simulink subsystem "PvtSubSys_PLAN_AP"  (R2020b)
settings: Solver=VariableStepAuto  StartTime=0.0  StopTime=10.0  RelTol=1e-3
undefined symbols (not defined in the file or in its folder): C_LongCtrl_0_Single, C_LongCtrl_0_Uint8, C_LongCtrl_Mph2Kph, magnitude, P_LongCtrl_accelTargAbsThrd, P_LongCtrl_AddVelAccelChange, P_LongCtrl_AddVelAccelThrd, P_LongCtrl_AddVelDistDesThrd, P_LongCtrl_AddVelEnable, P_LongCtrl_AddVelRefMsThrd, P_LongCtrl_ALaLowerChar, P_LongCtrl_ALaUpperCharEco, P_LongCtrl_ALaUpperCharNormal, P_LongCtrl_ALaUpperCharSport, P_LongCtrl_ALCAccLimitByDangerXAxis, P_LongCtrl_ALCAccLimitByDangerYAxis, P_LongCtrl_ALvAcceleLowerChar, P_LongCtrl_ALvAcceleUpperCharEco, P_LongCtrl_ALvAcceleUpperCharNormal, P_LongCtrl_ALvAcceleUpperCharSport, P_LongCtrl_CCaccelCCNeg2PosJerk, P_LongCtrl_CCaccelCCPosJerk, P_LongCtrl_CCaccelLowerIsLaneChange, P_LongCtrl_CCaccelMaxLCActive, P_LongCtrl_CCaccelMinECOAL, P_LongCtrl_CCaccelMinFastDecel, P_LongCtrl_CCaccelMinNoFastDecel, P_LongCtrl_CCaccelMinNormAL, P_LongCtrl_CCaccelMinSportAL, P_LongCtrl_CCaccelUpperCC, P_LongCtrl_CCaccelUpperCCSafeStop, P_LongCtrl_CCaMinNegAcceleLowerBand, P_LongCtrl_CCaMinNegAcceleUpperBand, P_LongCtrl_CCaMinPosAcceleLowerBand, P_LongCtrl_CCaMinPosAcceleUpperBand, P_LongCtrl_CCbECO, P_LongCtrl_CCbNorm, P_LongCtrl_CCbSport, P_LongCtrl_CCcoefESPSpd2IPSpd1, P_LongCtrl_CCcoefESPSpd2IPSpd2, P_LongCtrl_CCdecelCCJerk, P_LongCtrl_CCdecelCCJerkNegVLCInternalAcc, P_LongCtrl_CCfacNegAcceleLowerBand, P_LongCtrl_CCfacNegAcceleUpperBand, P_LongCtrl_CCfacPosAcceleLowerBand, P_LongCtrl_CCfacPosAcceleUpperBand, P_LongCtrl_CCkECO, P_LongCtrl_CCkNorm, P_LongCtrl_CCkSport, P_LongCtrl_CCLCIncSetSpdAdd, P_LongCtrl_CCLCIncSetSpdAddCntStartValue, P_LongCtrl_CCResumeDelayDeltaVel, P_LongCtrl_CCtAcceleTimeNeg, P_LongCtrl_CCtAcceleTimeNegCorrXAxis, P_LongCtrl_CCtAcceleTimeNegCorrYAxis, P_LongCtrl_CCtAcceleTimePos, P_LongCtrl_CCtAcceleTimePosCorrXAxis, P_LongCtrl_CCtAcceleTimePosCorrYAxis, P_LongCtrl_CCtStepVelPlan, P_LongCtrl_CCtTotVelPlan ... (+150)
libraries: simulink x62, TrueDurationTime x1
(part 6 of 7)

== stateflow chart PvtSubSys_PLAN_AP/AP/AP/IC/CurvatureOfMapCalc/Chart ==
  state velSubjLimMap = velSubjLimChar(LongCtrl_IC_EHRV2_CurMatrixLP) [function]
  state velDelta = velDeltaCalc(velSubjLimMap,velSubj) [function]
  state accelICCurvatureMapMatrix = accelICCurvatureMapPosCalc(velDelta) [function]
  state accelICCurvatureMapMatrix = accelICCurvatureMapNegCalc(velDelta) [function]
  state accelICCurvatureMapMatrix = accelICCurvatureMapDistExceed(LongCtrl_IC_EHRV2_CurDisMatrix,velDelta) [function]
  state distDesCurvatureMap = distDesCurvatureMapCalc(velDelta,accelICCurvatureMapMatrix) [function]
  (default) -> (junction 1)
  (junction 1) -> (junction 6) [order 1] : [LongCtrl_IC_EHRV2_CurMatrixSize>0&&(min(LongCtrl_IC_EHRV2_CurMatrixLP)<0.15)]
  (junction 1) -> (junction 10) [order 2] : {accelICCurvatureMapMatrix=repmat(single(16),1,10);}
  (junction 6) -> (junction 8) : {velSubjLimMap = velSubjLimChar(LongCtrl_IC_EHRV2_CurMatrixLP);
      |  velDelta = velDeltaCalc(velSubjLimMap,velSubj);
      |  accelICCurvatureMapMatrix=repmat(single(16),1,10);
      |  distDesCurvatureMap=repmat(single(500),1,10);
      |  i=uint8(1);}
  (junction 8) -> (junction 13) [order 1] : [i<=LongCtrl_IC_EHRV2_CurMatrixSize&&...
      |  abs(LongCtrl_IC_EHRV2_CurMatrixLP(1,i))<0.15]
  (junction 91) -> (junction 8) : {i=i+uint8(1);}
  (junction 8) -> (junction 36) [order 2]
  (junction 13) -> (junction 69)
  (junction 69) -> (junction 70) [order 1] : [velDelta(i)>0]
  (junction 69) -> (junction 55) [order 2] : {accelICCurvatureMapMatrix(1,i) = accelICCurvatureMapNegCalc(velDelta(1,i));
      |  distDesCurvatureMap(1,i) = distDesCurvatureMapCalc(velDelta(1,i),accelICCurvatureMapMatrix(1,i));}
  (junction 70) -> (junction 73) : {accelICCurvatureMapMatrix(1,i) = accelICCurvatureMapPosCalc(velDelta(1,i));}
  (junction 55) -> (junction 56) [order 1] : [distDesCurvatureMap(1,i)>LongCtrl_IC_EHRV2_CurDisMatrix(1,i)]
  (junction 55) -> (junction 57) [order 2] : {accelICCurvatureMapMatrix(1,i) =single(0.5);}
  (junction 56) -> (junction 58) : {accelICCurvatureMapMatrix(1,i) = accelICCurvatureMapDistExceed(LongCtrl_IC_EHRV2_CurDisMatrix(1,i),velDelta(1,i));
      |  accelICCurvatureMapMatrix(1,i) =max(single(-3.5),accelICCurvatureMapMatrix(1,i));}
  (junction 58) -> (junction 57)
  (junction 57) -> (junction 91)
  (junction 73) -> (junction 91)
  (junction 36) -> (junction 10)
  (junction 10) -> (junction 103) : {accelICCurvatureMapMin=min(accelICCurvatureMapMatrix);}
  (junction 103) -> (junction 107) [order 1] : [accelICCurvatureMapMin>0]
  (junction 103) -> (junction 111) [order 2] : {accelDesCurvatureMap=accelICCurvatureMapMin;}
  (junction 107) -> (junction 109) : {accelDesCurvatureMap=accelICCurvatureMapMatrix(1);}
  (junction 109) -> (junction 111)
  (junction 111) -> (junction 114)
  (junction 114) -> (junction 117) [order 1] : [P_LongCtrl_IC_EHRV2Enable==0]
  (junction 114) -> (junction 121) [order 2]
  (junction 117) -> (junction 119) : {accelDesCurvatureMap=single(16);}
  (junction 119) -> (junction 121)
  (junction 121) -> (junction 124)
  data: LongCtrl_IC_EHRV2_CurMatrixLP function_input single size=[1 10]; velSubjLimMap function_output; velSubjLimMap function_input single size=[1 10]; velSubj function_input single size=1; velDelta function_output; velDelta function_input single size=1; accelICCurvatureMapMatrix function_output; velDelta function_input single size=1; accelICCurvatureMapMatrix function_output; LongCtrl_IC_EHRV2_CurDisMatrix function_input single size=1; accelICCurvatureMapMatrix function_output; velDelta function_input single size=1; velDelta function_input single size=1; accelICCurvatureMapMatrix function_input single size=1; distDesCurvatureMap function_output; LongCtrl_IC_EHRV2_CurMatrixLP input single size=[1,10]; LongCtrl_IC_EHRV2_CurDisMatrix input single size=[1,10]; LongCtrl_IC_EHRV2_CurMatrixSize input uint8; velSubj input single; i local uint8; velSubjLimMap local single size=[1,10]; accelICCurvatureMapMatrix output single size=[1,10]; velDelta local single size=[1,10]; accelICCurvatureMapMin local single; distDesCurvatureMap output single size=[1,10]; accelDesCurvatureMap output single; P_LongCtrl_IC_EHRV2Enable parameter boolean

== stateflow chart PvtSubSys_PLAN_AP/AP/AP/IC/CurvatureOfRoadCalc/If Action Subsystem/For Each Subsystem/CurvatureChar ==
  state Curvature1 = Curvature1Calc(GetL1dC2V,GetL1dC3V,GetR1dC2V,GetR1dC3V,GetL1dDisFront,GetR1dDisFront,velSubj) [function]
  state Curvature2 = Curvature2Calc(GetL1dC2V,GetL1dC3V,GetL1dDisFront,velSubj) [function]
  state Curvature3 = Curvature3Calc(GetR1dC2V,GetR1dC3V,GetR1dDisFront,velSubj) [function]
  (default) -> (junction 10)
  (junction 10) -> (junction 12) [order 1] : [(L1bIsLineExist==1)&&(R1bIsLineExis==1)]
  (junction 10) -> (junction 11) [order 2]
  (junction 12) -> (junction 17) : {Curvature1 = Curvature1Calc(GetL1dC2V,GetL1dC3V,GetR1dC2V,GetR1dC3V,GetL1dDisFront,GetR1dDisFront,velSubj);
      |  CurvatureIFC=Curvature1;}
  (junction 11) -> (junction 29) [order 1] : [(L1bIsLineExist==1)&&(R1bIsLineExis!=1)]
  (junction 11) -> (junction 27) [order 2]
  (junction 29) -> (junction 36) : {Curvature2 = Curvature2Calc(GetL1dC2V,GetL1dC3V,GetL1dDisFront,velSubj);
      |  CurvatureIFC=Curvature2;}
  (junction 27) -> (junction 40) [order 1] : [(L1bIsLineExist!=1)&&(R1bIsLineExis==1)]
  (junction 27) -> (junction 38) [order 2] : {CurvatureIFC=single(0);}
  (junction 40) -> (junction 42) : {Curvature3 = Curvature3Calc(GetR1dC2V,GetR1dC3V,GetR1dDisFront,velSubj);
      |  CurvatureIFC=Curvature3;}
  data: GetL1dC2V function_input; GetL1dC3V function_input; GetR1dC2V function_input; GetR1dC3V function_input; GetL1dDisFront function_input; GetR1dDisFront function_input; Curvature1 function_output; velSubj function_input; GetL1dC2V function_input; GetL1dC3V function_input; GetL1dDisFront function_input; Curvature2 function_output; velSubj function_input; GetR1dC2V function_input; GetR1dC3V function_input; GetR1dDisFront function_input; Curvature3 function_output; velSubj function_input; L1bIsLineExist input boolean; R1bIsLineExis input boolean; CurvatureIFC output single; Curvature1 local double; Curvature2 local double; Curvature3 local double; GetL1dC2V input; GetL1dC3V input; GetL1dDisFront input; GetR1dC2V input; GetR1dC3V input; GetR1dDisFront input; velSubj input

== matlab function PvtSubSys_PLAN_AP/AP/AP/IC/Subsystem1/CalcEgoVehMove ==
  data: dDeltaX output single size=1; tCycle input single size=1; Kap input single size=1; velSubj input single size=1; dDeltaY output single size=1; CosOfPsi output single size=1; SinOfPsi output single size=1
function [dDeltaX,dDeltaY,CosOfPsi,SinOfPsi] = EgoVehicleMovement(tCycle,Kap,velSubj)
%#codegen
if Kap==0
    dDeltaX = velSubj*tCycle;
    dDeltaY = single(0);
    CosOfPsi = single(1);
    SinOfPsi = single(0);
else
    t_Psi = Kap*velSubj*tCycle;
    SinOfPsi = sin(t_Psi);
    CosOfPsi = cos(t_Psi);
    dDeltaX = SinOfPsi/Kap;
    dDeltaY = 2*(sin(t_Psi/2)*sin(t_Psi/2))/Kap;
end

== matlab function PvtSubSys_PLAN_AP/AP/AP/IC/Subsystem1/KeepLane ==
  data: KeepLineSts output; P_LongCtrl_KeepLaneTime input; P_LongCtrl_KeepLaneSurDis input; tCycle input single; velSubj input; Cur_LineValid input boolean; Cur_A3 input single; Cur_A2 input single; Cur_A1 input single; Cur_A0 input single; Cur_dDisFront input single; LineUpdate input boolean; dDeltaX input single; dDeltaY input single; CosOfPsi input single; SinOfPsi input single; LineValidK1 input boolean; A3K1 input single; A2K1 input single; A1K1 input single; A0K1 input single; dDisFrontK1 input single; tLostK1 input single; LineValid output boolean; A3 output single; A2 output single; A1 output single; A0 output single; dDisFront output single; tLost output single
function [KeepLineSts,LineValid,A3,A2,A1,A0,dDisFront,tLost] = ...
    VisFilter(P_LongCtrl_KeepLaneTime,P_LongCtrl_KeepLaneSurDis,...
    tCycle,velSubj,Cur_LineValid,Cur_A3,Cur_A2,Cur_A1,Cur_A0,Cur_dDisFront,LineUpdate,...
    dDeltaX,dDeltaY,CosOfPsi,SinOfPsi,...
    LineValidK1,A3K1,A2K1,A1K1,A0K1,dDisFrontK1,tLostK1)

A3 = single(zeros(2,1));
A2 = single(zeros(2,1));
A1 = single(zeros(2,1));
A0 = single(zeros(2,1));
dDisFront = single(zeros(2,1));
tLost = single(zeros(2,1));
LineValid = false(2,1);
KeepLineSts = uint8(zeros(2,1));
for i=1:1:2
    if (Cur_LineValid(i)==true)&&(LineUpdate==true)
        LineValid(i) = true;
        A3(i) = Cur_A3(i);
        A2(i) = Cur_A2(i);
        A1(i) = Cur_A1(i);
        A0(i) = Cur_A0(i);
        dDisFront(i) = Cur_dDisFront(i);
        tLost(i) = single(0);
        KeepLineSts(i) = uint8(0);
    else
        tLost(i) = min(tLostK1(i) + tCycle,single(10));
        if (LineValidK1(i)==true)&&(tLost(i)<P_LongCtrl_KeepLaneTime)
            xi = [0;0.25*dDisFrontK1(i);0.5*dDisFrontK1(i);dDisFrontK1(i)];
            yi = A3K1(i)*xi.^3 + A2K1(i)*xi.^2 + A1K1(i)*xi + A0K1(i);
            t_dx = xi-dDeltaX;
            t_dy = yi-dDeltaY;
            TmpX = t_dx*CosOfPsi+t_dy*SinOfPsi;
            TmpY = -t_dx*SinOfPsi+t_dy*CosOfPsi;
            [A3(i),A2(i),A1(i),A0(i)] = pl(TmpX,TmpY);
            LineValid(i) = true;
            dDisFront(i) = dDisFrontK1(i) - velSubj*tCycle;
            if dDisFront(i)<P_LongCtrl_KeepLaneSurDis
                LineValid(i) = false;
                KeepLineSts(i) = uint8(1);
            else
                KeepLineSts(i) = uint8(2);
            end
        else
            LineValid(i) = false;
            A3(i) = single(0);
            A2(i) = single(0);
            A1(i) = single(0);
            A0(i) = single(0);
            dDisFront(i) = single(0);
            KeepLineSts(i) = uint8(3);
        end
    end
end

== matlab function PvtSubSys_PLAN_AP/AP/AP/IC/Subsystem1/LineFilter ==
  data: P_LongCtrl_LaneAvailStd input; P_LongCtrl_LaneAvailStdMax input; P_LongCtrl_LaneAvailStdAverage input; A3 output single size=2; A2 output single size=2; A1 output single size=2; A0 output single size=2; tCycle input single size=1; bIsLineExis input uint8 size=2; a3 input single size=2; a2 input single size=2; a1 input single size=2; a0 input single size=2; dDeltaX input single size=1; velSubj input single size=1; A3K1 input single size=2; A2K1 input single size=2; A1K1 input single size=2; A0K1 input single size=2; Avail_timeK1 input single; Avail_disK1 input single; Avail_time output single; Avail_dis output single; Line_std output; Line_std_average input; Line_stdK1 input
function [A3,A2,A1,A0,Avail_time,Avail_dis,Line_std] = ...
    VisFilter(P_LongCtrl_LaneAvailStd,P_LongCtrl_LaneAvailStdMax,P_LongCtrl_LaneAvailStdAverage,tCycle,bIsLineExis,a3,a2,a1,a0,dDeltaX,velSubj,...
    A3K1,A2K1,A1K1,A0K1,Avail_timeK1,Avail_disK1,Line_std_average,Line_stdK1)

LaneConf = uint8(zeros(2,1));
A3 = single(zeros(2,1));
A2 = single(zeros(2,1));
A1 = single(zeros(2,1));
A0 = single(zeros(2,1));
Line_std = single(zeros(2,1));
Avail_time = Avail_timeK1;
Avail_dis = Avail_disK1;

for i=1:2
        LaneConf(i) = bIsLineExis(i);
        A3(i) = a3(i);
        A2(i) = a2(i);
        A1(i) = a1(i);
        A0(i) = a0(i);
end


%%  边界线校验
for i = 1:2
    if LaneConf(i)==single(2)
        t_Dist = max(single(15),single(3)*velSubj);
        xi = [single(0.05)*t_Dist;single(0.6)*t_Dist;single(0.8)*t_Dist;t_Dist];
        yi = A3K1(i)*xi.^single(3) + A2K1(i)*xi.^single(2) + A1K1(i)*xi + A0K1(i);
        t_dx = xi-dDeltaX;
        y = A3(i)*t_dx.^single(3)+A2(i)*t_dx.^single(2)+A1(i)*t_dx+A0(i);
        Error = y - yi;
        Line_std(i) = std(Error);
%         if Line_std(i)<P_LongCtrl_LaneAvailStd
        if (Line_stdK1(i)<P_LongCtrl_LaneAvailStd)||((Line_stdK1(i)<P_LongCtrl_LaneAvailStdMax)&&(Line_std_average(i)<P_LongCtrl_LaneAvailStdAverage))
            Avail_time(i) = min(Avail_timeK1(i)+tCycle,single(150));
            Avail_dis(i) = min(Avail_disK1(i)+tCycle*velSubj,single(150));
        else
            Avail_time(i) = single(0);
            Avail_dis(i) = single(0);
        end
    else 
        Avail_time(i) = single(0);
        Avail_dis(i) = single(0);
    end
end

== matlab function PvtSubSys_PLAN_AP/AP/AP/IC/AccelArbIC/MATLAB Function ==
  data: accelMap input single; accelCurvature input single; accelIC output single; accelKap input single; IC_state output uint8
function [accelIC,IC_state] = fcn(accelMap,accelCurvature,accelKap)
if  accelKap<=accelMap&&accelKap<=accelCurvature
    accelIC = accelKap;
    IC_state = uint8(2);
else
    accelIC = min(accelMap,accelCurvature);
    IC_state = uint8(1);
end

== stateflow chart PvtSubSys_PLAN_AP/AP/AP/ORD/ORD ==
  state [velDelta,IPKVel] = velDeltaCalc(velOffRampLimit,vehicleSpd) [function]
  state accelOffRamp = accelOffRampPosCalc(velDelta) [function]
  state accelOffRamp = accelOffRampNegCalc(velDelta) [function]
  state accelOffRamp = accelOffRampDistExceed(distRamp2Cur,StartVel,EndVel) [function]
  state distDesOffRamp = distDesOffRampCalc(StartVel,EndVel,accelOffRamp) [function]
  (default) -> (junction 1) : {[velDelta,IPKVel] = velDeltaCalc(velOffRampLimit,vehicleSpd);}
  (junction 1) -> (junction 3) [order 1] : [velOffRampLimit<255&&distRamp2Cur<2000&&...
      |  velDelta<P_LongCtrl_ORDvelDeltaEnableThres&&velOffRampLimit>1&&P_LongCtrl_ORDdecelEnable==1]
  (junction 1) -> (junction 43) [order 2] : {accelOffRamp=single(16);
      |  offRampDecelStart=false;}
  (junction 3) -> (junction 57)
  (junction 57) -> (junction 59) [order 1] : [velDelta>0]
  (junction 57) -> (junction 5) [order 2] : {accelOffRamp = accelOffRampNegCalc(velDelta);
      |  distDesOffRamp = distDesOffRampCalc(IPKVel,velOffRampLimit,accelOffRamp);}
  (junction 59) -> (junction 61) : {accelOffRamp = accelOffRampPosCalc(velDelta);}
  (junction 5) -> (junction 11) [order 1] : [distDesOffRamp>distRamp2Cur]
  (junction 5) -> (junction 90) [order 2]
  (junction 11) -> (junction 13) : {accelOffRamp = accelOffRampDistExceed(distRamp2Cur,IPKVel,velOffRampLimit);
      |  accelOffRamp =max(single(-3.5),accelOffRamp);}
  (junction 13) -> (junction 90)
  (junction 90) -> (junction 79)
  (junction 79) -> (junction 36) [order 1] : [(distDesOffRamp+single(30)>distRamp2Cur)||(offRampDecelStart==true)]
  (junction 79) -> (junction 34) [order 2] : {accelOffRamp=single(16);}
  (junction 36) -> (junction 38) : {offRampDecelStart=true;}
  (junction 38) -> (junction 34)
  (junction 34) -> (junction 40)
  (junction 40) -> (junction 43)
  (junction 61) -> (junction 40)
  (junction 43) -> (junction 46)
  data: velOffRampLimit function_input uint8 size=1; vehicleSpd function_input single size=1; velDelta function_output; IPKVel function_output; velDelta function_input single size=1; accelOffRamp function_output; velDelta function_input single size=1; accelOffRamp function_output; distRamp2Cur function_input uint16 size=1; accelOffRamp function_output; StartVel function_input single size=1; EndVel function_input uint8 size=1; StartVel function_input single size=1; EndVel function_input uint8 size=1; accelOffRamp function_input single size=1; distDesOffRamp function_output; vehicleSpd input; velOffRampLimit input; distRamp2Cur input; accelOffRamp output; distDesOffRamp local; velDelta local; offRampDecelStart local =false; P_LongCtrl_ORDdecelEnable parameter; P_LongCtrl_ORDvelDeltaEnableThres parameter; IPKVel local

== stateflow chart PvtSubSys_PLAN_AP/AP/AP/SJ/DeceleToStop/DeceleToStop ==
  state velTargetAbs = VxTargetCalc(velSubj,velTargetRel) [function]
  state distRes = DresCalc(distTargRel) [function]
  (default) -> (junction 1)
  (junction 1) -> (junction 12) [order 1] : [(ACCModeSts==3||ACCModeSts==4)&&...
      |  TargetExistP0==true]
  (junction 1) -> (junction 42) [order 2]
  (junction 12) -> (junction 14) : {velTargetAbs = VxTargetCalc(velSubj,velTargetRel);
      |  distRes = DresCalc(distTargRel);}
  (junction 42) -> (junction 44) [order 1] : [ACCModeSts==6||ACCModeSts==9]
  (junction 14) -> (junction 17) [order 1] : [(velTargetAbs<P_LongCtrl_velTargetThreDecleToStop)&&...
      |  (velSubj<P_LongCtrl_velSubjThreDecToStop)&&...
      |   distRes<distThreDecToStop]
  (junction 42) -> (junction 48) [order 2] : {DecleToStop=false;}
  (junction 44) -> (junction 46) : {DecleToStop=true;}
  (junction 14) -> (junction 30) [order 2]
  (junction 17) -> (junction 23) : {DecleToStop=true;}
  (junction 46) -> (junction 48)
  (junction 23) -> (junction 30)
  (junction 48) -> (junction 51)
  (junction 30) -> (junction 33)
  (junction 33) -> (junction 35) [order 1] : [VlcInternalAcc>C_LongCtrl_0_Single]
  (junction 33) -> (junction 39) [order 2]
  (junction 35) -> (junction 37) : {DecleToStop=false;}
  (junction 39) -> (junction 51)
  (junction 37) -> (junction 39)
  (junction 51) -> (junction 54)
  (junction 54) -> (junction 60) [order 1] : [DriveOffConditonFulfilled==true]
  (junction 54) -> (junction 64) [order 2]
  (junction 60) -> (junction 62) : {DecleToStop=false;}
  (junction 62) -> (junction 64)
  (junction 64) -> (junction 67)
  (junction 67) -> (junction 70) [order 1] : [velSubj<3&&SafeStopActive==1]
  (junction 67) -> (junction 74) [order 2]
  (junction 70) -> (junction 72) : {DecleToStop=true;}
  (junction 72) -> (junction 74)
  (junction 74) -> (junction 77)
  data: velSubj function_input single size=1; velTargetRel function_input single size=1; velTargetAbs function_output; distTargRel function_input single size=1; distRes function_output; velSubj input single; velTargetRel input single; velTargetAbs local; TargetExistP0 input boolean; ACCModeSts input uint8; P_LongCtrl_velTargetThreDecleToStop parameter; distRes local; C_LongCtrl_0_Single parameter; VlcInternalAcc input; DecleToStop output; distTargRel input; DriveOffConditonFulfilled input boolean; SafeStopActive input; distThreDecToStop input; P_LongCtrl_velSubjThreDecToStop parameter

== stateflow chart PvtSubSys_PLAN_AP/AP/AP/AL/AL ==
  (default) -> (junction 8)
  (junction 8) -> (junction 10) [order 1] : [DrivingMode==0]
  (junction 8) -> (junction 14) [order 2]
  (junction 10) -> (junction 12) : {ALAcceUpper=AcceUpperLimitNormalMode;}
  (junction 14) -> (junction 16) [order 1] : [DrivingMode==1]
  (junction 14) -> (junction 26) [order 2]
  (junction 16) -> (junction 21) : {ALAcceUpper=AcceUpperLimitSportMode;}
  (junction 26) -> (junction 28) [order 1] : [DrivingMode==6]
  (junction 26) -> (junction 62) [order 2] : {ALAcceUpper=AcceUpperLimitNormalMode;}
  (junction 28) -> (junction 30) : {ALAcceUpper=AcceUpperLimitEcoMode;}
  (junction 30) -> (junction 62)
  (junction 62) -> (junction 59)
  (junction 21) -> (junction 59)
  (junction 59) -> (junction 56)
  (junction 12) -> (junction 56)
  (junction 56) -> (junction 65)
  (junction 65) -> (junction 67) [order 1] : [HWASlowQuit==true]
  (junction 65) -> (junction 71) [order 2]
  (junction 67) -> (junction 69) : {ALAcceUpper=min(single(0),ALAcceUpper);}
  (junction 69) -> (junction 71)
  (junction 71) -> (junction 35) : {accelAL=max(AcceLowerLimit,min(accelArb,ALAcceUpper));
      |  upperBandAL=max(accelAL,min(upperBandArb,ALAcceUpper));
      |  lowerBandAL=max(AcceLowerLimit,min(accelAL,lowerBandArb));
      |  upperJerkAL=upperJerkArb;
      |  lowerJerkAL=lowerJerkArb;}
  data: accelAL output single; upperBandAL output single; AcceUpperLimitNormalMode input single; AcceUpperLimitSportMode input single; AcceUpperLimitEcoMode input single; AcceLowerLimit input single; DrivingMode input uint8; accelArb input single; ALAcceUpper local single; lowerBandAL output single; upperJerkAL output single; upperBandArb input single; lowerBandArb input single; lowerJerkAL output single; upperJerkArb input single; lowerJerkArb input single; HWASlowQuit input

== matlab function PvtSubSys_PLAN_AP/AP/AP/SJ/DisBar/ACC_DisplayBar1/ACC_DisplayBar ==
  data: TimeGap input; DisplayBar output uint8; DesireDistance input; ACCmode input; TargetRange input; Scale input; TargetExist input; DisplayBarK1 input uint8
function DisplayBar = fcn(TimeGap,DesireDistance,ACCmode,TargetRange,Scale,TargetExist,DisplayBarK1)
%#codegen
DisplayBar = uint8(DisplayBarK1);

ScaleDis = Scale*DesireDistance;
upScaleDis = (Scale+single(0.05))*DesireDistance;
lowScaleDis = (Scale-single(0.05))*DesireDistance;

i = TimeGap;

if (ACCmode==0)||(ACCmode==7)
    DisplayBar = uint8(0);
else
    if TargetExist==false
        DisplayBar=uint8(0);
    else
        switch(DisplayBarK1)
            case uint8(0)
                 if TargetRange> ScaleDis(i,3)
                     DisplayBar=uint8(4);
                 else
                     if TargetRange>ScaleDis(i,2)
                         DisplayBar=uint8(3);
                     else
                         if TargetRange>ScaleDis(i,1)
                             DisplayBar=uint8(2);
                         else
                             DisplayBar=uint8(1);
                         end
                     end
                 end
            case uint8(1)
                 if TargetRange> upScaleDis(i,3)
                     DisplayBar=uint8(4);
                 else
                     if TargetRange>upScaleDis(i,2)
                         DisplayBar=uint8(3);
                     else
                         if TargetRange>upScaleDis(i,1)
                             DisplayBar=uint8(2);
                         else
                             DisplayBar=uint8(1);
                         end
                     end
                 end
            case uint8(2)
                 if TargetRange> upScaleDis(i,3)
                     DisplayBar=uint8(4);
                 else
                     if TargetRange>upScaleDis(i,2)
                         DisplayBar=uint8(3);
                     else
                         if TargetRange>lowScaleDis(i,1)
                             DisplayBar=uint8(2);
                         else
                             DisplayBar=uint8(1);
                         end
                     end
                 end   
            case uint8(3)
                 if TargetRange> upScaleDis(i,3)
                     DisplayBar=uint8(4);
                 else
                     if TargetRange>lowScaleDis(i,2)
                         DisplayBar=uint8(3);
                     else
                         if TargetRange>lowScaleDis(i,1)
                             DisplayBar=uint8(2);
                         else
                             DisplayBar=uint8(1);
                         end
                     end
                end
            case uint8(4)
                 if TargetRange> lowScaleDis(i,3)
                     DisplayBar=uint8(4);
                 else
                     if TargetRange>lowScaleDis(i,2)
                         DisplayBar=uint8(3);
                     else
                         if TargetRange>lowScaleDis(i,1)
                             DisplayBar=uint8(2);
                         else
                             DisplayBar=uint8(1);
                         end
                     end
                 end      
        end    
    end
end

== stateflow chart PvtSubSys_PLAN_AP/AP/AP/SJ/DriverOffConditionFulfilled/DriveOff_Judge ==
  state Initialize
    entry:
    DriveOffConditonFulfilled=uint8(3);
  state DriveOff_Judge_TargetExist
    entry:
    velTargAbs=velSubj+velTargRel;
    DesiredDistGap=dDesired+P_LongCtrl_FollowDrvOffDistOffsetdDesiredAutoDrvOff;
    dxSensObj_modify=distTargRel;
    during:
    DriveOffConditonFulfilled=uint8(0);
    velTargAbs=velSubj+velTargRel;
    DesiredDistGap=dDesired+P_LongCtrl_FollowDrvOffDistOffsetdDesiredAutoDrvOff;
    dxSensObj_modify=distTargRel;
  state DriveOff_Follow
    entry:
    DriveOffConditonFulfilled=uint8(2);
    during:
    velTargAbs=velSubj+velTargRel;
    DesiredDistGap=dDesired+P_LongCtrl_FollowDrvOffDistOffsetdDesiredAutoDrvOff;
    dxSensObj_modify=distTargRel;
  state DriveOff_DisEnough
    entry:
    DriveOffConditonFulfilled=uint8(1);
    during:
    velTargAbs=velSubj+velTargRel;
    DesiredDistGap=dDesired+P_LongCtrl_FollowDrvOffDistOffsetdDesiredAutoDrvOff;
    dxSensObj_modify=distTargRel;
  (default) -> Initialize
  Initialize -> DriveOff_Judge_TargetExist
  DriveOff_Judge_TargetExist -> DriveOff_Follow [order 1] : [(velSubj<P_LongCtrl_FollowDrvOffStandstillVelThres)&&...
      | (velSet>P_LongCtrl_FollowDrvOffvSetMinDriveOffConditions)&&...
      | (targetExist==1)&&(ObjTypeP0~=uint8(6))&&...
      | (((velTargRel>P_LongCtrl_FollowDrvOffVelRelMinAutoDrvOff)&&(dxSensObj_modify>P_LongCtrl_FollowDrvOffdistRelMinAutoDrvOff))||...
      | ((ACCModeSts==5)&&(velTargRel>(P_LongCtrl_FollowDrvOffVelRelMinAutoDrvOff-P_LongCtrl_FollowDrvOffVelCorrVelFullFillOverride))&&(dxSensObj_modify>(P_LongCtrl_FollowDrvOffdistRelMinAutoDrvOff-P_LongCtrl_FollowDrvOffDistCorrVelFullFillOverride))))]
  (junction 59) -> DriveOff_Follow [order 1] : [(velSubj<P_LongCtrl_FollowDrvOffStandstillVelThres)&&...
      | (velSet>P_LongCtrl_FollowDrvOffvSetMinDriveOffConditions)&&...
      | (targetExist==1)&&...
      | (((velTargRel>P_LongCtrl_FollowDrvOffVelRelMinAutoDrvOff)&&(dxSensObj_modify>P_LongCtrl_FollowDrvOffdistRelMinAutoDrvOff))||...
      | ((ACCModeSts==5)&&(velTargRel>(P_LongCtrl_FollowDrvOffVelRelMinAutoDrvOff-P_LongCtrl_FollowDrvOffVelCorrVelFullFillOverride))&&...
      | (dxSensObj_modify>(P_LongCtrl_FollowDrvOffdistRelMinAutoDrvOff-P_LongCtrl_FollowDrvOffDistCorrVelFullFillOverride))))]
  DriveOff_Follow -> (junction 56) : [(velSubj>=P_LongCtrl_FollowDrvOffStandstillVelThres)||...
      | (velSet<=P_LongCtrl_FollowDrvOffvSetMinDriveOffConditions)||...
      | (targetExist==0)||...
      | ((targetExist==1)&&...
      | (((ACCModeSts~=5)&&((velTargRel<=(P_LongCtrl_FollowDrvOffVelRelMinAutoDrvOff-P_LongCtrl_FollowDrvOffVelExitVelCorrNoOverride))||(dxSensObj_modify<=(P_LongCtrl_FollowDrvOffdistRelMinAutoDrvOff-P_LongCtrl_FollowDrvOffVelExitDistCorrNoOverride))))||...
      | ((ACCModeSts==5)&&((velTargRel<=(P_LongCtrl_FollowDrvOffVelRelMinAutoDrvOff-P_LongCtrl_FollowDrvOffVelExitVelCorrOverride))||(dxSensObj_modify<=(P_LongCtrl_FollowDrvOffdistRelMinAutoDrvOff-P_LongCtrl_FollowDrvOffVelExitDistCorrOverride))))))]
  (junction 59) -> DriveOff_Judge_TargetExist [order 2]
  DriveOff_Judge_TargetExist -> DriveOff_DisEnough [order 2] : [(velSubj<P_LongCtrl_FollowDrvOffStandstillVelThres)&&...
      | (velSet>P_LongCtrl_FollowDrvOffvSetMinDriveOffConditions)&&...
      | ((targetExist==0)||...
      | ((targetExist==1)&&(ObjTypeP0~=uint8(6))&&(dxSensObj_modify>DesiredDistGap))||...
      | ((ACCModeSts==5)&&(targetExist==1)&&(dxSensObj_modify>(DesiredDistGap-P_LongCtrl_FollowDrvOffDistCorrDistFullFillOverride))))]
  (junction 56) -> DriveOff_Judge_TargetExist [order 2]
  DriveOff_DisEnough -> (junction 59) : [(velSubj>=P_LongCtrl_FollowDrvOffStandstillVelThres)||...
      | (velSet<=P_LongCtrl_FollowDrvOffvSetMinDriveOffConditions)||...
      | ((ACCModeSts~=5)&&(targetExist==1)&&(dxSensObj_modify<=(DesiredDistGap-P_LongCtrl_FollowDrvOffDistExitNoOverride)))||...
      | ((ACCModeSts==5)&&(targetExist==1)&&(dxSensObj_modify<=(DesiredDistGap-P_LongCtrl_FollowDrvOffDistExitOverride)))]
  (junction 56) -> DriveOff_DisEnough [order 1] : [(velSubj<P_LongCtrl_FollowDrvOffStandstillVelThres)&&...
      | (velSet>P_LongCtrl_FollowDrvOffvSetMinDriveOffConditions)&&...
      | ((targetExist==0)||...
      | ((targetExist==1)&&(dxSensObj_modify>DesiredDistGap))||...
      | ((ACCModeSts==5)&&(targetExist==1)&&(dxSensObj_modify>(DesiredDistGap-P_LongCtrl_FollowDrvOffDistCorrDistFullFillOverride))))]
  data: velSubj input single; dDesired input single; velSet input single; velTargRel input single; distTargRel input single; targetExist input boolean; DriveOffConditonFulfilled output uint8; DesiredDistGap local single; P_LongCtrl_FollowDrvOffStandstillVelThres parameter single; P_LongCtrl_FollowDrvOffDistOffsetdDesiredAutoDrvOff parameter single; P_LongCtrl_FollowDrvOffdistRelMinAutoDrvOff parameter single; P_LongCtrl_FollowDrvOffVelRelMinAutoDrvOff parameter single; P_LongCtrl_FollowDrvOffvSetMinDriveOffConditions parameter single; dxSensObj_modify local single; velTargAbs local single; ACCModeSts input; P_LongCtrl_FollowDrvOffDistCorrDistFullFillOverride parameter; P_LongCtrl_FollowDrvOffVelCorrVelFullFillOverride parameter; P_LongCtrl_FollowDrvOffDistCorrVelFullFillOverride parameter; P_LongCtrl_FollowDrvOffDistExitNoOverride parameter; P_LongCtrl_FollowDrvOffDistExitOverride parameter; P_LongCtrl_FollowDrvOffVelExitVelCorrNoOverride parameter; P_LongCtrl_FollowDrvOffVelExitDistCorrNoOverride parameter; P_LongCtrl_FollowDrvOffVelExitVelCorrOverride parameter; P_LongCtrl_FollowDrvOffVelExitDistCorrOverride parameter; ObjTypeP0 input

== matlab function PvtSubSys_PLAN_AP/AP/AP/Subsystem/MATLAB Function ==
  data: u input; ACCModeSts output; Counter input single; CounterK1 output single
function [ACCModeSts,CounterK1] = fcn(u,Counter)
if (u(1)==7)&&((u(2)==6)||u(2)==(9))
    Counter=single(76);
end
if Counter>0
    ACCModeSts=uint8(6);
    CounterK1=max(single(0),Counter-single(1));
else
    ACCModeSts = u(1);
    CounterK1=single(0);
end

== stateflow chart PvtSubSys_PLAN_AP/AP/AP/FollowCtrl/AccelSupression/AccelSupression ==
  state NoAutoLaneChange
    en:
    accelRelEnter=max(single(0.1),accelTargAbsEnable-P_LongCtrl_FollowaccelMinAccelSupressionEnter);
    distAccelSupressionMinEnter=velTargRel^2/(single(2)*accelRelEnter)+velSubj*single(0.4);
    accelSupressionEnable=false;
    during:
    accelRelEnter=max(single(0.1),accelTargAbsEnable-P_LongCtrl_FollowaccelMinAccelSupressionEnter);
    distAccelSupressionMinEnter=velTargRel^2/(single(2)*accelRelEnter)+velSubj*single(0.4);
  state AutoLaneChange
    en:
    accelRelExit=max(single(0.1),accelTargAbsEnable-P_LongCtrl_FollowaccelMinAccelSupressionExit);
    distAccelSupressionMinExit=velTargRel^2/(single(2)*accelRelExit)+velSubj*single(0.4);
    during:
    accelRelExit=max(single(0.1),accelTargAbsEnable-P_LongCtrl_FollowaccelMinAccelSupressionExit);
    distAccelSupressionMinExit=velTargRel^2/(single(2)*accelRelExit)+velSubj*single(0.4);
    accelSupressionEnable=true;
  (default) -> NoAutoLaneChange
  NoAutoLaneChange -> AutoLaneChange : [(laneChangeEnable==1)&&...
      | (accelTargAbsEnable>-2)&&...
      | (distTargRel>distAccelSupressionMinEnter)&&...
      | (dangerLevel<=P_LongCtrl_DangerLevelEnterThrd)]
  AutoLaneChange -> NoAutoLaneChange : [(laneChangeEnable~=1)||...
      | (accelTargAbsEnable<=-2)||...
      | (distTargRel<=distAccelSupressionMinExit)||...
      | (dangerLevel>P_LongCtrl_DangerLevelExitThrd)]
  data: velTargRel input; accelTargAbsEnable input; velSubj input; laneChangeEnable input; distTargRel input; accelSupressionEnable output; P_LongCtrl_FollowaccelMinAccelSupressionEnter input; P_LongCtrl_FollowaccelMinAccelSupressionExit input; accelRelEnter local; accelRelExit local; distAccelSupressionMinEnter output; distAccelSupressionMinExit output; P_LongCtrl_DangerLevelEnterThrd input single size=[1 1]; P_LongCtrl_DangerLevelExitThrd input single size=[1 1]; dangerLevel input single size=[1 1]

== stateflow chart PvtSubSys_PLAN_AP/AP/AP/VlcInternalAccCalc/Chart ==
  (default) -> (junction 1)
  (junction 1) -> (junction 3) [order 1] : [(ACCModeSts(1)==3)&&(ACCModeSts(2)~=3)]
  (junction 1) -> (junction 7) [order 2] : {tNoneActive2Active=max(single(0),tNoneActive2Active-tCycle);}
  (junction 3) -> (junction 5) : {tNoneActive2Active=single(0.4);}
  (junction 5) -> (junction 7)
  (junction 7) -> (junction 16)
  (junction 16) -> (junction 18) [order 1] : [ACCModeSts(1)~=3]
  (junction 16) -> (junction 22) [order 2]
  (junction 18) -> (junction 20) : {tNoneActive2Active=single(0);}
  (junction 20) -> (junction 22)
  (junction 22) -> (junction 25) : {VlcAcc=accelSubj*(tNoneActive2Active/0.4)+VlcInternalAcc*(0.4-tNoneActive2Active)/0.4;}
  data: ACCModeSts input; tCycle input; tNoneActive2Active local =single(0); VlcInternalAcc input; accelSubj input; VlcAcc output

== matlab function PvtSubSys_PLAN_AP/AP/AP/CCCtrl/MATLAB Function ==
  data: LCAIncSetSpdReq input; SetSpd output; ACCSetSpd input; ACCSetSpdK1 input; SpdIncValue input; CntStartValue input; CntK1 input uint8; Cnt output; P_LongCtrl_CCLCIncSetSpdEnable parameter boolean
function [SetSpd,Cnt] = fcn(LCAIncSetSpdReq,ACCSetSpd,ACCSetSpdK1,SpdIncValue,CntStartValue, CntK1, P_LongCtrl_CCLCIncSetSpdEnable)
if CntK1 > 0
    Cnt = CntK1 - uint8(1);
else
    Cnt = CntK1;
end
if (LCAIncSetSpdReq==uint8(1))&&(P_LongCtrl_CCLCIncSetSpdEnable==true)
   Cnt = uint8(CntStartValue); 
end
if ACCSetSpd~=ACCSetSpdK1
    Cnt = uint8(0); 
end
t = single(Cnt)/single(CntStartValue);
SetSpd = t * SpdIncValue + ACCSetSpd;

== stateflow chart PvtSubSys_PLAN_AP/AP/AP/SJ/TakeOver/Chart ==
  state TorCtrlOnCounter
    en:
    Cnt = 1;
    TorCtrlReq = 0;
    du:
    Cnt = Cnt + 1;
  state TorCtrlOff
    en:
    Cnt = 1;
    TorCtrlReq = 0;
  state TorCtrlOn
    en:
    Cnt = 1;
    TorCtrlReq = 1;
  (default) -> TorCtrlOff
  TorCtrlOff -> TorCtrlOnCounter : [distRelPlanMin<P_LongCtrl_FollowcoefDistRelThresActiveTOR*distRelDesDistRelPlanNumMin]
  TorCtrlOnCounter -> TorCtrlOff [order 1] : [distRelPlanMin>P_LongCtrl_FollowcoefDistRelThresActiveTOR*distRelDesDistRelPlanNumMin]
  TorCtrlOn -> TorCtrlOff : [distRelPlanMin>P_LongCtrl_FollowcoefDistRelThresActiveTOR*distRelDesDistRelPlanNumMin]
  TorCtrlOnCounter -> TorCtrlOn [order 2] : [(distRelPlanMin<P_LongCtrl_FollowcoefDistRelThresActiveTOR*distRelDesDistRelPlanNumMin)&&...
      | Cnt>WaitSteps]
  data: WaitSteps input; Cnt output; TorCtrlReq output; distRelPlanMin input; distRelDesDistRelPlanNumMin input; P_LongCtrl_FollowcoefDistRelThresActiveTOR parameter

== stateflow chart PvtSubSys_PLAN_AP/AP/AP/SJ/TakeOver/TakeOver ==
  (default) -> (junction 1)
  (junction 1) -> (junction 3) [order 1] : [((ACCModeSts==3)&&(targetExistP0==true))&&...
      |  (((gap<P_LongCtrl_FollowgapThresActiveTOR)&&(accelFollow<P_LongCtrl_FollowaccelThresActiveTOR))||...
      |  ((TorCtrlReq==1)&&(velTargetRel<P_LongCtrl_FollowvelTargRelThresActiveTOR)))]
  (junction 1) -> (junction 7) [order 2] : {tor=false;}
  (junction 3) -> (junction 5) : {tor=true;}
  (junction 5) -> (junction 7)
  (junction 7) -> (junction 18)
  data: ACCModeSts input uint8; gap input single; accelFollow input single; targetExistP0 input boolean; velTargetRel input single; tor output boolean; P_LongCtrl_FollowgapThresActiveTOR parameter; P_LongCtrl_FollowaccelThresActiveTOR parameter; P_LongCtrl_FollowcoefDistRelThresActiveTOR parameter; P_LongCtrl_FollowvelTargRelThresActiveTOR parameter; TorCtrlReq input

== stateflow chart PvtSubSys_PLAN_AP/AP/AP/CCCtrl/velPlanCC/Chart ==
  (default) -> (junction 1) : {i=uint8(1);
      |  iMax=uint8(P_LongCtrl_CCtTotVelPlan/P_LongCtrl_CCtStepVelPlan);
      |  velSubjPlanCC=velSubj;
      |  accelPlanStepCur=VLCInternalAccK1;
      |  velSubjPlanCC2ALC=single(zeros(1,8));}
  (junction 1) -> (junction 3) [order 1] : [i<=iMax]
  (junction 5) -> (junction 1)
  (junction 1) -> (junction 9) [order 2]
  (junction 3) -> (junction 94)
  (junction 94) -> (junction 83) [order 1] : [drivingMode==0]
  (junction 94) -> (junction 85) [order 2]
  (junction 83) -> (junction 89) : {accelMaxAL=max(P_LongCtrl_CCaccelMinNormAL,(velSubjPlanCC*P_LongCtrl_CCkNorm+P_LongCtrl_CCbNorm));}
  (junction 89) -> (junction 85)
  (junction 85) -> (junction 104)
  (junction 104) -> (junction 99) [order 1] : [drivingMode==1]
  (junction 104) -> (junction 82) [order 2]
  (junction 99) -> (junction 97) : {accelMaxAL=max(P_LongCtrl_CCaccelMinSportAL,(velSubjPlanCC*P_LongCtrl_CCkSport+P_LongCtrl_CCbSport));}
  (junction 97) -> (junction 82)
  (junction 82) -> (junction 81)
  (junction 81) -> (junction 90) [order 1] : [drivingMode==6]
  (junction 81) -> (junction 92) [order 2]
  (junction 90) -> (junction 93) : {accelMaxAL=max(P_LongCtrl_CCaccelMinECOAL,(velSubjPlanCC*P_LongCtrl_CCkECO+P_LongCtrl_CCbECO));}
  (junction 93) -> (junction 92)
  (junction 92) -> (junction 24)
  (junction 24) -> (junction 26) [order 1] : [fastDecel==true]
  (junction 24) -> (junction 30) [order 2] : {accelMinAL=P_LongCtrl_CCaccelMinNoFastDecel;}
  (junction 26) -> (junction 28) : {accelMinAL=P_LongCtrl_CCaccelMinFastDecel;}
  (junction 28) -> (junction 30)
  (junction 30) -> (junction 13)
  (junction 13) -> (junction 15) [order 1] : [accelCCLim>=accelPlanStepCur&&accelPlanStepCur<=0]
  (junction 13) -> (junction 33) [order 2]
  (junction 15) -> (junction 17) : {accelPlanStepNext=min(min(accelCCLim,accelMaxAL),(accelPlanStepCur+...
      | P_LongCtrl_CCtStepVelPlan*P_LongCtrl_CCaccelCCNeg2PosJerk));}
  (junction 33) -> (junction 34) [order 1] : [accelCCLim>=accelPlanStepCur&&accelPlanStepCur>=0]
  (junction 33) -> (junction 43) [order 2]
  (junction 34) -> (junction 36) : {accelPlanStepNext=min(min(accelCCLim,accelMaxAL),(accelPlanStepCur+...
      | P_LongCtrl_CCtStepVelPlan*P_LongCtrl_CCaccelCCPosJerk));}
  (junction 43) -> (junction 45) [order 1] : [accelCCLim<=accelPlanStepCur&&accelPlanStepCur>=0]
  (junction 43) -> (junction 49) [order 2] : {accelPlanStepNext=max(max(accelCCLim,accelMinAL),(accelPlanStepCur+...
      | P_LongCtrl_CCtStepVelPlan*P_LongCtrl_CCdecelCCJerkNegVLCInternalAcc));}
  (junction 45) -> (junction 47) : {accelPlanStepNext=max(max(accelCCLim,accelMinAL),(accelPlanStepCur+...
      | P_LongCtrl_CCtStepVelPlan*P_LongCtrl_CCdecelCCJerk));}
  (junction 47) -> (junction 49)
  (junction 49) -> (junction 38)
  (junction 36) -> (junction 38)
  (junction 38) -> (junction 19)
  (junction 17) -> (junction 19)
  (junction 19) -> (junction 5) : {accelPlanStepAver=(accelPlanStepNext+accelPlanStepCur)/single(2);
      |  velSubjPlanCC=velSubjPlanCC+P_LongCtrl_CCtStepVelPlan*accelPlanStepAver;
      |  accelPlanStepCur=accelPlanStepNext;
      |  velSubjPlanCC2ALC(1,i)=velSubjPlanCC;
      |  i=i+uint8(1);}
  data: drivingMode input; i local; iMax local; velSubjPlanCC local; accelPlanStepNext local; accelPlanStepCur local; accelPlanStepAver local; accelMaxAL local; accelMinAL local; velSubjPlanCC2ALC output; velSubj input; fastDecel input; accelCCLim input; VLCInternalAccK1 input; P_LongCtrl_CCdecelCCJerkNegVLCInternalAcc input; P_LongCtrl_CCdecelCCJerk input; P_LongCtrl_CCaccelMinNoFastDecel input; P_LongCtrl_CCaccelMinFastDecel input; P_LongCtrl_CCtTotVelPlan input; P_LongCtrl_CCtStepVelPlan input; P_LongCtrl_CCaccelCCNeg2PosJerk input; P_LongCtrl_CCaccelCCPosJerk input; P_LongCtrl_CCaccelMinECOAL input; P_LongCtrl_CCaccelMinSportAL input; P_LongCtrl_CCaccelMinNormAL input; P_LongCtrl_CCbNorm input; P_LongCtrl_CCkNorm input; P_LongCtrl_CCbECO input; P_LongCtrl_CCkECO input; P_LongCtrl_CCbSport input; P_LongCtrl_CCkSport input

== stateflow chart PvtSubSys_PLAN_AP/AP/AP/Arbitrate/Arbitrate ==
  (default) -> (junction 38) : {velPlanEffect=uint8(0);}
  (junction 38) -> (junction 39) [order 1] : [ACCModeSts==3||...
      | ACCModeSts==4||...
      | ACCModeSts==5||...
      | ACCModeSts==6||...
      | ACCModeSts==9]
  (junction 38) -> (junction 42) [order 2] : {accelArb=C_LongCtrl_0_Single;
      |  upperBandArb=C_LongCtrl_0_Single;
      |  lowerBandArb=C_LongCtrl_0_Single;
      |  upperJerkArb=C_LongCtrl_0_Single;
      |  lowerJerkArb=C_LongCtrl_0_Single;}
  (junction 39) -> (junction 1)
  (junction 1) -> (junction 3) [order 1] : [targetExistP0==true]
  (junction 1) -> (junction 47) [order 2]
  (junction 3) -> (junction 19)
  (junction 19) -> (junction 21) [order 1] : [accelFollow<accelCC]
  (junction 19) -> (junction 56) [order 2]
  (junction 21) -> (junction 65)
  (junction 47) -> (junction 49) [order 1] : [accelCC<accelIC]
  (junction 56) -> (junction 58) [order 1] : [accelCC<accelIC]
  (junction 65) -> (junction 67) [order 1] : [accelFollow<accelIC]
  (junction 47) -> (junction 53) [order 2] : {accelArb=accelIC;
      |  upperBandArb=upperBandIC;
      |  lowerBandArb=lowerBandIC;
      |  upperJerkArb=upperJerkIC;
      |  lowerJerkArb=lowerJerkIC;
      |  ArbFlag=uint8(2);}
  (junction 49) -> (junction 51) : {accelArb=accelCC;
      |  upperBandArb=upperBandCC;
      |  lowerBandArb=lowerBandCC;
      |  upperJerkArb=upperJerkCC;
      |  lowerJerkArb=lowerJerkCC;
      |  ArbFlag=uint8(1);}
  (junction 56) -> (junction 62) [order 2] : {accelArb=accelIC;
      |  upperBandArb=upperBandIC;
      |  lowerBandArb=lowerBandIC;
      |  upperJerkArb=upperJerkIC;
      |  lowerJerkArb=lowerJerkIC;
      |  ArbFlag=uint8(2);}
  (junction 58) -> (junction 60) : {accelArb=accelCC;
      |  upperBandArb=upperBandCC;
      |  lowerBandArb=lowerBandCC;
      |  upperJerkArb=upperJerkCC;
      |  lowerJerkArb=lowerJerkCC;
      |  ArbFlag=uint8(1);}
  (junction 65) -> (junction 71) [order 2] : {accelArb=accelIC;
      |  upperBandArb=upperBandIC;
      |  lowerBandArb=lowerBandIC;
      |  upperJerkArb=upperJerkIC;
      |  lowerJerkArb=lowerJerkIC;
      |  ArbFlag=uint8(2);}
  (junction 67) -> (junction 69) : {accelArb=accelFollow;
      |  upperBandArb=upperBandFollow;
      |  lowerBandArb=lowerBandFollow;
      |  upperJerkArb=upperJerkFollow;
      |  lowerJerkArb=lowerJerkFollow;
      |  ArbFlag=uint8(4);}
  (junction 51) -> (junction 53)
  (junction 60) -> (junction 62)
  (junction 69) -> (junction 71)
  (junction 53) -> (junction 5)
  (junction 62) -> (junction 25)
  (junction 71) -> (junction 23)
  (junction 25) -> (junction 5)
  (junction 23) -> (junction 25)
  (junction 5) -> (junction 80)
  (junction 80) -> (junction 82) [order 1] : [accelArb<accelORD]
  (junction 80) -> (junction 86) [order 2] : {accelArb=accelORD;
      |  upperBandArb=upperBandORD;
      |  lowerBandArb=lowerBandORD;
      |  upperJerkArb=upperJerkORD;
      |  lowerJerkArb=lowerJerkORD;
      |  ArbFlag=uint8(3);}
  (junction 82) -> (junction 84)
  (junction 84) -> (junction 86)
  (junction 86) -> (junction 104)
  (junction 104) -> (junction 106) [order 1] : [ArbFlag==1]
  (junction 104) -> (junction 110) [order 2]
  (junction 106) -> (junction 108) : {accelArb=accelCCCtrlAfterJerk;
      |  velPlanEffect=uint8(1);}
  (junction 110) -> (junction 115) [order 1] : [ArbFlag==4]
  (junction 110) -> (junction 120) [order 2]
  (junction 115) -> (junction 117) : {accelArb=accelFollowAfterJerk;
      |  velPlanEffect=uint8(2);}
  (junction 120) -> (junction 42)
  (junction 117) -> (junction 120)
  (junction 108) -> (junction 117)
  (junction 42) -> (junction 90)
  data: accelCC input single; lowerBandCC input single; upperBandCC input single; lowerJerkCC input single; upperJerkCC input single; accelCCCtrlAfterJerk input; accelIC input; upperBandIC input; lowerBandIC input; upperJerkIC input; lowerJerkIC input; accelORD input; upperBandORD input; lowerBandORD input; upperJerkORD input; lowerJerkORD input; accelArb output single; lowerBandArb output single; lowerJerkArb output single; upperBandArb output single; upperJerkArb output single; accelFollow input single; accelFollowAfterJerk input; upperBandFollow input single; lowerBandFollow input single; upperJerkFollow input single; lowerJerkFollow input single; targetExistP0 input boolean; ACCModeSts input uint8; C_LongCtrl_0_Single parameter; velPlanEffect output uint8; ArbFlag output double

== stateflow chart PvtSubSys_PLAN_AP/AP/AP/CCCtrl/AccelCCCalc ==
  state accelCC = CCAccelePos(deltaVelCC) [function]
  state accelCC = CCAcceleNeg(deltaVelCC) [function]
  state deltaVelCC= CCDeltaVCalc(CCSetSpd,VehicleSpd) [function]
  state ACC_SpdSetValueMph2Kph = Mph2KphCalc(SpdSetValue) [function]
  (default) -> (junction 65) : {SpdSetValue=ACC_SpdSetValue;}
  (junction 65) -> (junction 66) [order 1] : [SafeStopActive==1]
  (junction 65) -> (junction 70) [order 2]
  (junction 66) -> (junction 68) : {SpdSetValue=single(0);}
  (junction 68) -> (junction 70)
  (junction 70) -> (junction 3)
  (junction 3) -> (junction 6) [order 1] : [IP_VehSpdUnit==C_LongCtrl_0_Uint8]
  (junction 3) -> (junction 8) [order 2] : {ACC_SpdSetValueMph2Kph = Mph2KphCalc(SpdSetValue);
      | CCSetSpd=ACC_SpdSetValueMph2Kph;}
  (junction 6) -> (junction 10) : {CCSetSpd=SpdSetValue;}
  (junction 10) -> (junction 8)
  (junction 8) -> (junction 16) : {deltaVelCC = CCDeltaVCalc(CCSetSpd,VehicleSpd);}
  (junction 16) -> (junction 21) [order 1] : [deltaVelCC>C_LongCtrl_0_Single]
  (junction 16) -> (junction 28) [order 2] : {accelCC = CCAcceleNeg(deltaVelCC);}
  (junction 21) -> (junction 23) : {accelCC = CCAccelePos(deltaVelCC);}
  (junction 23) -> (junction 28)
  (junction 28) -> (junction 37)
  (junction 37) -> (junction 44) [order 1] : [((CCSetSpd<CCSetSpdK1)&&(deltaVelCC<(P_LongCtrl_CCResumeDelayDeltaVel)))||vSetBelowMin==1||SafeStopActive==1]
  (junction 37) -> (junction 53) [order 2]
  (junction 44) -> (junction 46) : {fastDecel=true;}
  (junction 53) -> (junction 54) [order 1] : [(deltaVelCC>(-1))&&(SafeStopActive==0)]
  (junction 53) -> (junction 58) [order 2]
  (junction 54) -> (junction 56) : {fastDecel=false;}
  (junction 56) -> (junction 58)
  (junction 58) -> (junction 48)
  (junction 46) -> (junction 48)
  (junction 48) -> (junction 51) : {CCSetSpdK1=CCSetSpd;}
  data: deltaVelCC function_input single size=1; accelCC function_output single; deltaVelCC function_input single size=1; accelCC function_output single; CCSetSpd function_input single size=1; VehicleSpd function_input single size=1; deltaVelCC function_output; SpdSetValue function_input single size=1; ACC_SpdSetValueMph2Kph function_output single; ACC_SpdSetValue input single; VehicleSpd input single; IP_VehSpdUnit input uint8; C_LongCtrl_0_Uint8 parameter; CCSetSpd local single; C_LongCtrl_0_Single parameter; accelCC output single; deltaVelCC local single; ACC_SpdSetValueMph2Kph local single; CCSetSpdK1 local double =single(255); fastDecel output double =false; vSetBelowMin input; SafeStopActive input; SpdSetValue local double; P_LongCtrl_CCResumeDelayDeltaVel parameter single

== stateflow chart PvtSubSys_PLAN_AP/AP/AP/CCCtrl/AcceleBandCC ==
  state [upperBandCC,lowerBandCC] = CCPosAcceleBandCalc(accelCCDes) [function]
  state [upperBandCC,lowerBandCC] = CCNegAcceleBandCalc(accelCCDes) [function]
  (default) -> (junction 39)
  (junction 39) -> (junction 42) [order 1] : [accelCCDes>C_LongCtrl_0_Single]
  (junction 39) -> (junction 51) [order 2] : {[upperBandCC,lowerBandCC] = CCNegAcceleBandCalc(accelCCDes);}
  (junction 42) -> (junction 45) : {[upperBandCC,lowerBandCC] = CCPosAcceleBandCalc(accelCCDes);}
  (junction 45) -> (junction 51)
  (junction 51) -> (junction 58)
  data: accelCCDes function_input single size=1; upperBandCC function_output single; lowerBandCC function_output single; accelCCDes function_input single size=1; upperBandCC function_output single; lowerBandCC function_output single; accelCCDes input single; C_LongCtrl_0_Single parameter single; lowerBandCC output; upperBandCC output

== matlab function PvtSubSys_PLAN_AP/AP/AP/FollowCtrl/AccelSupression/DecelJudge ==
  data: accelSubjPlanOpt input; tStartDecel output; IDP0 input; P_LongCtrl_FollowaccelSupressionAccelThres parameter single
function tStartDecel = fcn(accelSubjPlanOpt,IDP0, P_LongCtrl_FollowaccelSupressionAccelThres)
tStartDecel=single(100);
if IDP0~=0
     for i=1:40
            if accelSubjPlanOpt(i)<P_LongCtrl_FollowaccelSupressionAccelThres
               tStartDecel=single(0.5)*(single(i)-single(1));break; 
            end
     end
end

== matlab function PvtSubSys_PLAN_AP/AP/AP/FollowCtrl/PlausibilityCheck/PlausibilityCheck ==
  data: FollowAccele input single; velSubj input single; FollowAccele_Plau output single; velTargAbs input single; distRelPlanTerminate input single; num input single; IDP0 input; FollowAcceleK1 input single; PlauCheckEnable output; distTargRel input; P_LongCtrl_FollowvelSubjThresEnablePlauCheck parameter; P_LongCtrl_FollowvelRelThresEnablePlauCheck parameter; P_LongCtrl_FollowvelSubjMaxEnablePlauCheck parameter; P_LongCtrl_FollowdistRelThresEnablePlauCheck parameter; P_LongCtrl_FollowdistRelDevCalcDistConst parameter; P_LongCtrl_FollowcoefAccelFadeOutPlauCheck parameter
function [FollowAccele_Plau,PlauCheckEnable]= fcn(FollowAccele,velSubj,velTargAbs,distRelPlanTerminate,num,IDP0,FollowAcceleK1,distTargRel, P_LongCtrl_FollowvelSubjThresEnablePlauCheck, P_LongCtrl_FollowvelRelThresEnablePlauCheck, P_LongCtrl_FollowvelSubjMaxEnablePlauCheck, P_LongCtrl_FollowdistRelThresEnablePlauCheck, P_LongCtrl_FollowdistRelDevCalcDistConst, P_LongCtrl_FollowcoefAccelFadeOutPlauCheck)
velRel=velTargAbs-velSubj;
accelConst=single(255);
if (velSubj>P_LongCtrl_FollowvelSubjThresEnablePlauCheck)&&(velRel<P_LongCtrl_FollowvelRelThresEnablePlauCheck)&&(velSubj<P_LongCtrl_FollowvelSubjMaxEnablePlauCheck)&&(distTargRel<P_LongCtrl_FollowdistRelThresEnablePlauCheck)
   accelConst= -((velTargAbs-velSubj)^2)/(single(2)*max(single(0.1),distRelPlanTerminate(1,num)-P_LongCtrl_FollowdistRelDevCalcDistConst));
end
if (accelConst<FollowAccele)&&(FollowAccele<-0.3)
    if (FollowAcceleK1<FollowAccele)&&(IDP0(1)==IDP0(2))&&(IDP0(2)~=0)
        FollowAccele_Plau=FollowAcceleK1*P_LongCtrl_FollowcoefAccelFadeOutPlauCheck;
        PlauCheckEnable=true;
    else
        FollowAccele_Plau=FollowAccele;
        PlauCheckEnable=false;
    end
else
    FollowAccele_Plau=FollowAccele;
    PlauCheckEnable=false;
end
